simulink model "correlator_core"  (Simulink 7.1)
settings: Solver=ode45  StartTime=0.0  StopTime=10000  RelTol=1e-3
libraries: xbsIndex_r4 x658, cfa_library x168, casper_library_delays x4, casper_library_misc x2
(part 2 of 9)

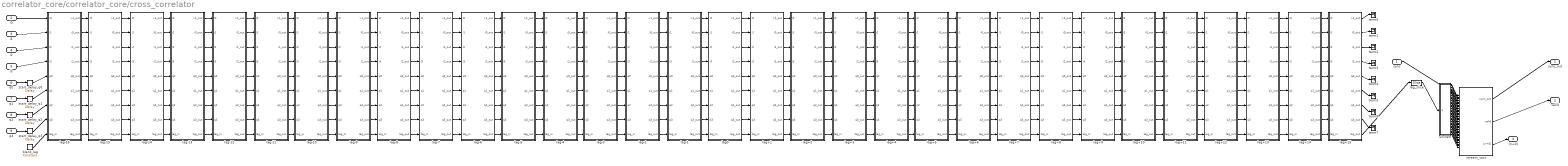
== system correlator_core/correlator_core/cross_correlator ==
  sync : Inport
  i0 : Inport  Port=2
  i1 : Inport  Port=3
  i2 : Inport  Port=4
  i3 : Inport  Port=5
  q0 : Inport  Port=6
  q1 : Inport  Port=7
  q2 : Inport  Port=8
  q3 : Inport  Port=9
  blank_lag : xbsIndex_r4/Constant  arith_type=Unsigned  const=0  n_bits=1  bin_pt=0  explicit_period=on  period=1  equ=P=C  opselect=C  inp2=PCIN>>17  opr=+  inp1=P  carry=CIN  dbl_ovrd=off  block_type=constant
      settings: block_version=11.4
  lag+1 : Subsystem  AncestorBlock=cfa_library/single_lag  mask(single_lag){n_inputs=2, specify_mult=off, mult_spec=Behavioral, specify_add=off, add_spec=Fabric, mult_delay=3, add_delay=2, overall_delay=2, use_2bit=on, shift_q=off, shift_i=on}
      mask prompts: n_inputs "Number of Simultaneous Inputs: (2^?)"; specify_mult "Specify multiplier use (behavioural HDL if not specified)"; mult_spec "Multiplier specification:"; specify_add "Specify adder use (behavioural HDL if not specified)"; add_spec "Adder specification:"; mult_delay "Mult Latency:"; add_delay "Add Latency:"; overall_delay "Overall Latency:"; use_2bit "Use special 2-bit binary encoding"; shift_q "Shift 'q' output"; shift_i "Shift 'i' output"
      mask help: This performs the computations for a single lag. Please use the 'cross_correlator' block to generate a full X-engine.
      mask init:
      | single_lag_init(gcb,...
      |     'n_inputs', n_inputs,...
      |     'specify_mult', specify_mult,...
      |     'mult_spec', mult_spec,...
      |     'specify_add', specify_add,...
      |     'add_spec', add_spec,...
      |     'mult_delay', mult_delay,...
      |     'add_delay', add_delay,...
      |     'overall_delay', overall_delay,...
      |     'use_2bit', use_2bit,...
      |     'shift_q', shift_q,...
      |     'shift_i', shift_i);
      settings: AttributesFormatString=|
      | Use 2-bit: on, Demux: 4,
      | Mult: Behavioral,
      | Add: Fabric
      mask StyleString: edit,checkbox,popup(Behavioral|Core|Embedded),checkbox,popup(Fabric|DSP48),edit,edit,edit,checkbox,checkbox,checkbox
      mask CallbackString:
      | |specify_mult = get_param(gcb,'specify_mult');
      | enables = get_param(gcb, 'MaskEnables');
      | if( strcmp(specify_mult,'off')),
      |     enables{3} = 'off';
      | else,
      |     enables{3} = 'on';
      | end
      | set_param(gcb, 'MaskEnables', enables);
      | ||specify_add = get_param(gcb,'specify_add');
      | enables = get_param(gcb, 'MaskEnables');
      | if( strcmp(specify_add,'off')),
      |     enables{5} = 'off';
      | else,
      |     enables{5} = 'on';
      | end
      | set_param(gcb, 'MaskEnables', enables);
      | |||||||
      mask TabNameString: Basic,Implementation,Implementation,Implementation,Implementation,Implementation,Implementation,Implementation,Basic,Basic,Basic
  lag+10 : Subsystem  AncestorBlock=cfa_library/single_lag  mask(single_lag){n_inputs=2, specify_mult=off, mult_spec=Behavioral, specify_add=off, add_spec=Fabric, mult_delay=3, add_delay=2, overall_delay=2, use_2bit=on, shift_q=off, shift_i=on}
      mask prompts: n_inputs "Number of Simultaneous Inputs: (2^?)"; specify_mult "Specify multiplier use (behavioural HDL if not specified)"; mult_spec "Multiplier specification:"; specify_add "Specify adder use (behavioural HDL if not specified)"; add_spec "Adder specification:"; mult_delay "Mult Latency:"; add_delay "Add Latency:"; overall_delay "Overall Latency:"; use_2bit "Use special 2-bit binary encoding"; shift_q "Shift 'q' output"; shift_i "Shift 'i' output"
      mask help: This performs the computations for a single lag. Please use the 'cross_correlator' block to generate a full X-engine.
      mask init: same as correlator_core/correlator_core/cross_correlator/lag+1
      settings: AttributesFormatString=|
      | Use 2-bit: on, Demux: 4,
      | Mult: Behavioral,
      | Add: Fabric
      mask StyleString: edit,checkbox,popup(Behavioral|Core|Embedded),checkbox,popup(Fabric|DSP48),edit,edit,edit,checkbox,checkbox,checkbox
      mask CallbackString:
      | |specify_mult = get_param(gcb,'specify_mult');
      | enables = get_param(gcb, 'MaskEnables');
      | if( strcmp(specify_mult,'off')),
      |     enables{3} = 'off';
      | else,
      |     enables{3} = 'on';
      | end
      | set_param(gcb, 'MaskEnables', enables);
      | ||specify_add = get_param(gcb,'specify_add');
      | enables = get_param(gcb, 'MaskEnables');
      | if( strcmp(specify_add,'off')),
      |     enables{5} = 'off';
      | else,
      |     enables{5} = 'on';
      | end
      | set_param(gcb, 'MaskEnables', enables);
      | |||||||
      mask TabNameString: Basic,Implementation,Implementation,Implementation,Implementation,Implementation,Implementation,Implementation,Basic,Basic,Basic
  lag+11 : Subsystem  AncestorBlock=cfa_library/single_lag  mask(single_lag){n_inputs=2, specify_mult=off, mult_spec=Behavioral, specify_add=off, add_spec=Fabric, mult_delay=3, add_delay=2, overall_delay=2, use_2bit=on, shift_q=off, shift_i=on}
      mask prompts: n_inputs "Number of Simultaneous Inputs: (2^?)"; specify_mult "Specify multiplier use (behavioural HDL if not specified)"; mult_spec "Multiplier specification:"; specify_add "Specify adder use (behavioural HDL if not specified)"; add_spec "Adder specification:"; mult_delay "Mult Latency:"; add_delay "Add Latency:"; overall_delay "Overall Latency:"; use_2bit "Use special 2-bit binary encoding"; shift_q "Shift 'q' output"; shift_i "Shift 'i' output"
      mask help: This performs the computations for a single lag. Please use the 'cross_correlator' block to generate a full X-engine.
      mask init: same as correlator_core/correlator_core/cross_correlator/lag+1
      settings: AttributesFormatString=|
      | Use 2-bit: on, Demux: 4,
      | Mult: Behavioral,
      | Add: Fabric
      mask StyleString: edit,checkbox,popup(Behavioral|Core|Embedded),checkbox,popup(Fabric|DSP48),edit,edit,edit,checkbox,checkbox,checkbox
      mask CallbackString:
      | |specify_mult = get_param(gcb,'specify_mult');
      | enables = get_param(gcb, 'MaskEnables');
      | if( strcmp(specify_mult,'off')),
      |     enables{3} = 'off';
      | else,
      |     enables{3} = 'on';
      | end
      | set_param(gcb, 'MaskEnables', enables);
      | ||specify_add = get_param(gcb,'specify_add');
      | enables = get_param(gcb, 'MaskEnables');
      | if( strcmp(specify_add,'off')),
      |     enables{5} = 'off';
      | else,
      |     enables{5} = 'on';
      | end
      | set_param(gcb, 'MaskEnables', enables);
      | |||||||
      mask TabNameString: Basic,Implementation,Implementation,Implementation,Implementation,Implementation,Implementation,Implementation,Basic,Basic,Basic
  lag+12 : Subsystem  AncestorBlock=cfa_library/single_lag  mask(single_lag){n_inputs=2, specify_mult=off, mult_spec=Behavioral, specify_add=off, add_spec=Fabric, mult_delay=3, add_delay=2, overall_delay=2, use_2bit=on, shift_q=off, shift_i=on}
      mask prompts: n_inputs "Number of Simultaneous Inputs: (2^?)"; specify_mult "Specify multiplier use (behavioural HDL if not specified)"; mult_spec "Multiplier specification:"; specify_add "Specify adder use (behavioural HDL if not specified)"; add_spec "Adder specification:"; mult_delay "Mult Latency:"; add_delay "Add Latency:"; overall_delay "Overall Latency:"; use_2bit "Use special 2-bit binary encoding"; shift_q "Shift 'q' output"; shift_i "Shift 'i' output"
      mask help: This performs the computations for a single lag. Please use the 'cross_correlator' block to generate a full X-engine.
      mask init: same as correlator_core/correlator_core/cross_correlator/lag+1
      settings: AttributesFormatString=|
      | Use 2-bit: on, Demux: 4,
      | Mult: Behavioral,
      | Add: Fabric
      mask StyleString: edit,checkbox,popup(Behavioral|Core|Embedded),checkbox,popup(Fabric|DSP48),edit,edit,edit,checkbox,checkbox,checkbox
      mask CallbackString:
      | |specify_mult = get_param(gcb,'specify_mult');
      | enables = get_param(gcb, 'MaskEnables');
      | if( strcmp(specify_mult,'off')),
      |     enables{3} = 'off';
      | else,
      |     enables{3} = 'on';
      | end
      | set_param(gcb, 'MaskEnables', enables);
      | ||specify_add = get_param(gcb,'specify_add');
      | enables = get_param(gcb, 'MaskEnables');
      | if( strcmp(specify_add,'off')),
      |     enables{5} = 'off';
      | else,
      |     enables{5} = 'on';
      | end
      | set_param(gcb, 'MaskEnables', enables);
      | |||||||
      mask TabNameString: Basic,Implementation,Implementation,Implementation,Implementation,Implementation,Implementation,Implementation,Basic,Basic,Basic
  lag+13 : Subsystem  AncestorBlock=cfa_library/single_lag  mask(single_lag){n_inputs=2, specify_mult=off, mult_spec=Behavioral, specify_add=off, add_spec=Fabric, mult_delay=3, add_delay=2, overall_delay=2, use_2bit=on, shift_q=off, shift_i=on}
      mask prompts: n_inputs "Number of Simultaneous Inputs: (2^?)"; specify_mult "Specify multiplier use (behavioural HDL if not specified)"; mult_spec "Multiplier specification:"; specify_add "Specify adder use (behavioural HDL if not specified)"; add_spec "Adder specification:"; mult_delay "Mult Latency:"; add_delay "Add Latency:"; overall_delay "Overall Latency:"; use_2bit "Use special 2-bit binary encoding"; shift_q "Shift 'q' output"; shift_i "Shift 'i' output"
      mask help: This performs the computations for a single lag. Please use the 'cross_correlator' block to generate a full X-engine.
      mask init: same as correlator_core/correlator_core/cross_correlator/lag+1
      settings: AttributesFormatString=|
      | Use 2-bit: on, Demux: 4,
      | Mult: Behavioral,
      | Add: Fabric
      mask StyleString: edit,checkbox,popup(Behavioral|Core|Embedded),checkbox,popup(Fabric|DSP48),edit,edit,edit,checkbox,checkbox,checkbox
      mask CallbackString:
      | |specify_mult = get_param(gcb,'specify_mult');
      | enables = get_param(gcb, 'MaskEnables');
      | if( strcmp(specify_mult,'off')),
      |     enables{3} = 'off';
      | else,
      |     enables{3} = 'on';
      | end
      | set_param(gcb, 'MaskEnables', enables);
      | ||specify_add = get_param(gcb,'specify_add');
      | enables = get_param(gcb, 'MaskEnables');
      | if( strcmp(specify_add,'off')),
      |     enables{5} = 'off';
      | else,
      |     enables{5} = 'on';
      | end
      | set_param(gcb, 'MaskEnables', enables);
      | |||||||
      mask TabNameString: Basic,Implementation,Implementation,Implementation,Implementation,Implementation,Implementation,Implementation,Basic,Basic,Basic
  lag+14 : Subsystem  AncestorBlock=cfa_library/single_lag  mask(single_lag){n_inputs=2, specify_mult=off, mult_spec=Behavioral, specify_add=off, add_spec=Fabric, mult_delay=3, add_delay=2, overall_delay=2, use_2bit=on, shift_q=off, shift_i=on}
      mask prompts: n_inputs "Number of Simultaneous Inputs: (2^?)"; specify_mult "Specify multiplier use (behavioural HDL if not specified)"; mult_spec "Multiplier specification:"; specify_add "Specify adder use (behavioural HDL if not specified)"; add_spec "Adder specification:"; mult_delay "Mult Latency:"; add_delay "Add Latency:"; overall_delay "Overall Latency:"; use_2bit "Use special 2-bit binary encoding"; shift_q "Shift 'q' output"; shift_i "Shift 'i' output"
      mask help: This performs the computations for a single lag. Please use the 'cross_correlator' block to generate a full X-engine.
      mask init: same as correlator_core/correlator_core/cross_correlator/lag+1
      settings: AttributesFormatString=|
      | Use 2-bit: on, Demux: 4,
      | Mult: Behavioral,
      | Add: Fabric
      mask StyleString: edit,checkbox,popup(Behavioral|Core|Embedded),checkbox,popup(Fabric|DSP48),edit,edit,edit,checkbox,checkbox,checkbox
      mask CallbackString:
      | |specify_mult = get_param(gcb,'specify_mult');
      | enables = get_param(gcb, 'MaskEnables');
      | if( strcmp(specify_mult,'off')),
      |     enables{3} = 'off';
      | else,
      |     enables{3} = 'on';
      | end
      | set_param(gcb, 'MaskEnables', enables);
      | ||specify_add = get_param(gcb,'specify_add');
      | enables = get_param(gcb, 'MaskEnables');
      | if( strcmp(specify_add,'off')),
      |     enables{5} = 'off';
      | else,
      |     enables{5} = 'on';
      | end
      | set_param(gcb, 'MaskEnables', enables);
      | |||||||
      mask TabNameString: Basic,Implementation,Implementation,Implementation,Implementation,Implementation,Implementation,Implementation,Basic,Basic,Basic
  lag+15 : Subsystem  AncestorBlock=cfa_library/single_lag  mask(single_lag){n_inputs=2, specify_mult=off, mult_spec=Behavioral, specify_add=off, add_spec=Fabric, mult_delay=3, add_delay=2, overall_delay=2, use_2bit=on, shift_q=off, shift_i=on}
      mask prompts: n_inputs "Number of Simultaneous Inputs: (2^?)"; specify_mult "Specify multiplier use (behavioural HDL if not specified)"; mult_spec "Multiplier specification:"; specify_add "Specify adder use (behavioural HDL if not specified)"; add_spec "Adder specification:"; mult_delay "Mult Latency:"; add_delay "Add Latency:"; overall_delay "Overall Latency:"; use_2bit "Use special 2-bit binary encoding"; shift_q "Shift 'q' output"; shift_i "Shift 'i' output"
      mask help: This performs the computations for a single lag. Please use the 'cross_correlator' block to generate a full X-engine.
      mask init: same as correlator_core/correlator_core/cross_correlator/lag+1
      settings: AttributesFormatString=|
      | Use 2-bit: on, Demux: 4,
      | Mult: Behavioral,
      | Add: Fabric
      mask StyleString: edit,checkbox,popup(Behavioral|Core|Embedded),checkbox,popup(Fabric|DSP48),edit,edit,edit,checkbox,checkbox,checkbox
      mask CallbackString:
      | |specify_mult = get_param(gcb,'specify_mult');
      | enables = get_param(gcb, 'MaskEnables');
      | if( strcmp(specify_mult,'off')),
      |     enables{3} = 'off';
      | else,
      |     enables{3} = 'on';
      | end
      | set_param(gcb, 'MaskEnables', enables);
      | ||specify_add = get_param(gcb,'specify_add');
      | enables = get_param(gcb, 'MaskEnables');
      | if( strcmp(specify_add,'off')),
      |     enables{5} = 'off';
      | else,
      |     enables{5} = 'on';
      | end
      | set_param(gcb, 'MaskEnables', enables);
      | |||||||
      mask TabNameString: Basic,Implementation,Implementation,Implementation,Implementation,Implementation,Implementation,Implementation,Basic,Basic,Basic
  lag+2 : Subsystem  AncestorBlock=cfa_library/single_lag  mask(single_lag){n_inputs=2, specify_mult=off, mult_spec=Behavioral, specify_add=off, add_spec=Fabric, mult_delay=3, add_delay=2, overall_delay=2, use_2bit=on, shift_q=off, shift_i=on}
      mask prompts: n_inputs "Number of Simultaneous Inputs: (2^?)"; specify_mult "Specify multiplier use (behavioural HDL if not specified)"; mult_spec "Multiplier specification:"; specify_add "Specify adder use (behavioural HDL if not specified)"; add_spec "Adder specification:"; mult_delay "Mult Latency:"; add_delay "Add Latency:"; overall_delay "Overall Latency:"; use_2bit "Use special 2-bit binary encoding"; shift_q "Shift 'q' output"; shift_i "Shift 'i' output"
      mask help: This performs the computations for a single lag. Please use the 'cross_correlator' block to generate a full X-engine.
      mask init: same as correlator_core/correlator_core/cross_correlator/lag+1
      settings: AttributesFormatString=|
      | Use 2-bit: on, Demux: 4,
      | Mult: Behavioral,
      | Add: Fabric
      mask StyleString: edit,checkbox,popup(Behavioral|Core|Embedded),checkbox,popup(Fabric|DSP48),edit,edit,edit,checkbox,checkbox,checkbox
      mask CallbackString:
      | |specify_mult = get_param(gcb,'specify_mult');
      | enables = get_param(gcb, 'MaskEnables');
      | if( strcmp(specify_mult,'off')),
      |     enables{3} = 'off';
      | else,
      |     enables{3} = 'on';
      | end
      | set_param(gcb, 'MaskEnables', enables);
      | ||specify_add = get_param(gcb,'specify_add');
      | enables = get_param(gcb, 'MaskEnables');
      | if( strcmp(specify_add,'off')),
      |     enables{5} = 'off';
      | else,
      |     enables{5} = 'on';
      | end
      | set_param(gcb, 'MaskEnables', enables);
      | |||||||
      mask TabNameString: Basic,Implementation,Implementation,Implementation,Implementation,Implementation,Implementation,Implementation,Basic,Basic,Basic
  lag+3 : Subsystem  AncestorBlock=cfa_library/single_lag  mask(single_lag){n_inputs=2, specify_mult=off, mult_spec=Behavioral, specify_add=off, add_spec=Fabric, mult_delay=3, add_delay=2, overall_delay=2, use_2bit=on, shift_q=off, shift_i=on}
      mask prompts: n_inputs "Number of Simultaneous Inputs: (2^?)"; specify_mult "Specify multiplier use (behavioural HDL if not specified)"; mult_spec "Multiplier specification:"; specify_add "Specify adder use (behavioural HDL if not specified)"; add_spec "Adder specification:"; mult_delay "Mult Latency:"; add_delay "Add Latency:"; overall_delay "Overall Latency:"; use_2bit "Use special 2-bit binary encoding"; shift_q "Shift 'q' output"; shift_i "Shift 'i' output"
      mask help: This performs the computations for a single lag. Please use the 'cross_correlator' block to generate a full X-engine.
      mask init: same as correlator_core/correlator_core/cross_correlator/lag+1
      settings: AttributesFormatString=|
      | Use 2-bit: on, Demux: 4,
      | Mult: Behavioral,
      | Add: Fabric
      mask StyleString: edit,checkbox,popup(Behavioral|Core|Embedded),checkbox,popup(Fabric|DSP48),edit,edit,edit,checkbox,checkbox,checkbox
      mask CallbackString:
      | |specify_mult = get_param(gcb,'specify_mult');
      | enables = get_param(gcb, 'MaskEnables');
      | if( strcmp(specify_mult,'off')),
      |     enables{3} = 'off';
      | else,
      |     enables{3} = 'on';
      | end
      | set_param(gcb, 'MaskEnables', enables);
      | ||specify_add = get_param(gcb,'specify_add');
      | enables = get_param(gcb, 'MaskEnables');
      | if( strcmp(specify_add,'off')),
      |     enables{5} = 'off';
      | else,
      |     enables{5} = 'on';
      | end
      | set_param(gcb, 'MaskEnables', enables);
      | |||||||
      mask TabNameString: Basic,Implementation,Implementation,Implementation,Implementation,Implementation,Implementation,Implementation,Basic,Basic,Basic
  lag+4 : Subsystem  AncestorBlock=cfa_library/single_lag  mask(single_lag){n_inputs=2, specify_mult=off, mult_spec=Behavioral, specify_add=off, add_spec=Fabric, mult_delay=3, add_delay=2, overall_delay=2, use_2bit=on, shift_q=off, shift_i=on}
      mask prompts: n_inputs "Number of Simultaneous Inputs: (2^?)"; specify_mult "Specify multiplier use (behavioural HDL if not specified)"; mult_spec "Multiplier specification:"; specify_add "Specify adder use (behavioural HDL if not specified)"; add_spec "Adder specification:"; mult_delay "Mult Latency:"; add_delay "Add Latency:"; overall_delay "Overall Latency:"; use_2bit "Use special 2-bit binary encoding"; shift_q "Shift 'q' output"; shift_i "Shift 'i' output"
      mask help: This performs the computations for a single lag. Please use the 'cross_correlator' block to generate a full X-engine.
      mask init: same as correlator_core/correlator_core/cross_correlator/lag+1
      settings: AttributesFormatString=|
      | Use 2-bit: on, Demux: 4,
      | Mult: Behavioral,
      | Add: Fabric
      mask StyleString: edit,checkbox,popup(Behavioral|Core|Embedded),checkbox,popup(Fabric|DSP48),edit,edit,edit,checkbox,checkbox,checkbox
      mask CallbackString:
      | |specify_mult = get_param(gcb,'specify_mult');
      | enables = get_param(gcb, 'MaskEnables');
      | if( strcmp(specify_mult,'off')),
      |     enables{3} = 'off';
      | else,
      |     enables{3} = 'on';
      | end
      | set_param(gcb, 'MaskEnables', enables);
      | ||specify_add = get_param(gcb,'specify_add');
      | enables = get_param(gcb, 'MaskEnables');
      | if( strcmp(specify_add,'off')),
      |     enables{5} = 'off';
      | else,
      |     enables{5} = 'on';
      | end
      | set_param(gcb, 'MaskEnables', enables);
      | |||||||
      mask TabNameString: Basic,Implementation,Implementation,Implementation,Implementation,Implementation,Implementation,Implementation,Basic,Basic,Basic
  lag+5 : Subsystem  AncestorBlock=cfa_library/single_lag  mask(single_lag){n_inputs=2, specify_mult=off, mult_spec=Behavioral, specify_add=off, add_spec=Fabric, mult_delay=3, add_delay=2, overall_delay=2, use_2bit=on, shift_q=off, shift_i=on}
      mask prompts: n_inputs "Number of Simultaneous Inputs: (2^?)"; specify_mult "Specify multiplier use (behavioural HDL if not specified)"; mult_spec "Multiplier specification:"; specify_add "Specify adder use (behavioural HDL if not specified)"; add_spec "Adder specification:"; mult_delay "Mult Latency:"; add_delay "Add Latency:"; overall_delay "Overall Latency:"; use_2bit "Use special 2-bit binary encoding"; shift_q "Shift 'q' output"; shift_i "Shift 'i' output"
      mask help: This performs the computations for a single lag. Please use the 'cross_correlator' block to generate a full X-engine.
      mask init: same as correlator_core/correlator_core/cross_correlator/lag+1
      settings: AttributesFormatString=|
      | Use 2-bit: on, Demux: 4,
      | Mult: Behavioral,
      | Add: Fabric
      mask StyleString: edit,checkbox,popup(Behavioral|Core|Embedded),checkbox,popup(Fabric|DSP48),edit,edit,edit,checkbox,checkbox,checkbox
      mask CallbackString:
      | |specify_mult = get_param(gcb,'specify_mult');
      | enables = get_param(gcb, 'MaskEnables');
      | if( strcmp(specify_mult,'off')),
      |     enables{3} = 'off';
      | else,
      |     enables{3} = 'on';
      | end
      | set_param(gcb, 'MaskEnables', enables);
      | ||specify_add = get_param(gcb,'specify_add');
      | enables = get_param(gcb, 'MaskEnables');
      | if( strcmp(specify_add,'off')),
      |     enables{5} = 'off';
      | else,
      |     enables{5} = 'on';
      | end
      | set_param(gcb, 'MaskEnables', enables);
      | |||||||
      mask TabNameString: Basic,Implementation,Implementation,Implementation,Implementation,Implementation,Implementation,Implementation,Basic,Basic,Basic
  lag+6 : Subsystem  AncestorBlock=cfa_library/single_lag  mask(single_lag){n_inputs=2, specify_mult=off, mult_spec=Behavioral, specify_add=off, add_spec=Fabric, mult_delay=3, add_delay=2, overall_delay=2, use_2bit=on, shift_q=off, shift_i=on}
      mask prompts: n_inputs "Number of Simultaneous Inputs: (2^?)"; specify_mult "Specify multiplier use (behavioural HDL if not specified)"; mult_spec "Multiplier specification:"; specify_add "Specify adder use (behavioural HDL if not specified)"; add_spec "Adder specification:"; mult_delay "Mult Latency:"; add_delay "Add Latency:"; overall_delay "Overall Latency:"; use_2bit "Use special 2-bit binary encoding"; shift_q "Shift 'q' output"; shift_i "Shift 'i' output"
      mask help: This performs the computations for a single lag. Please use the 'cross_correlator' block to generate a full X-engine.
      mask init: same as correlator_core/correlator_core/cross_correlator/lag+1
      settings: AttributesFormatString=|
      | Use 2-bit: on, Demux: 4,
      | Mult: Behavioral,
      | Add: Fabric
      mask StyleString: edit,checkbox,popup(Behavioral|Core|Embedded),checkbox,popup(Fabric|DSP48),edit,edit,edit,checkbox,checkbox,checkbox
      mask CallbackString:
      | |specify_mult = get_param(gcb,'specify_mult');
      | enables = get_param(gcb, 'MaskEnables');
      | if( strcmp(specify_mult,'off')),
      |     enables{3} = 'off';
      | else,
      |     enables{3} = 'on';
      | end
      | set_param(gcb, 'MaskEnables', enables);
      | ||specify_add = get_param(gcb,'specify_add');
      | enables = get_param(gcb, 'MaskEnables');
      | if( strcmp(specify_add,'off')),
      |     enables{5} = 'off';
      | else,
      |     enables{5} = 'on';
      | end
      | set_param(gcb, 'MaskEnables', enables);
      | |||||||
      mask TabNameString: Basic,Implementation,Implementation,Implementation,Implementation,Implementation,Implementation,Implementation,Basic,Basic,Basic
  lag+7 : Subsystem  AncestorBlock=cfa_library/single_lag  mask(single_lag){n_inputs=2, specify_mult=off, mult_spec=Behavioral, specify_add=off, add_spec=Fabric, mult_delay=3, add_delay=2, overall_delay=2, use_2bit=on, shift_q=off, shift_i=on}
      mask prompts: n_inputs "Number of Simultaneous Inputs: (2^?)"; specify_mult "Specify multiplier use (behavioural HDL if not specified)"; mult_spec "Multiplier specification:"; specify_add "Specify adder use (behavioural HDL if not specified)"; add_spec "Adder specification:"; mult_delay "Mult Latency:"; add_delay "Add Latency:"; overall_delay "Overall Latency:"; use_2bit "Use special 2-bit binary encoding"; shift_q "Shift 'q' output"; shift_i "Shift 'i' output"
      mask help: This performs the computations for a single lag. Please use the 'cross_correlator' block to generate a full X-engine.
      mask init: same as correlator_core/correlator_core/cross_correlator/lag+1
      settings: AttributesFormatString=|
      | Use 2-bit: on, Demux: 4,
      | Mult: Behavioral,
      | Add: Fabric
      mask StyleString: edit,checkbox,popup(Behavioral|Core|Embedded),checkbox,popup(Fabric|DSP48),edit,edit,edit,checkbox,checkbox,checkbox
      mask CallbackString:
      | |specify_mult = get_param(gcb,'specify_mult');
      | enables = get_param(gcb, 'MaskEnables');
      | if( strcmp(specify_mult,'off')),
      |     enables{3} = 'off';
      | else,
      |     enables{3} = 'on';
      | end
      | set_param(gcb, 'MaskEnables', enables);
      | ||specify_add = get_param(gcb,'specify_add');
      | enables = get_param(gcb, 'MaskEnables');
      | if( strcmp(specify_add,'off')),
      |     enables{5} = 'off';
      | else,
      |     enables{5} = 'on';
      | end
      | set_param(gcb, 'MaskEnables', enables);
      | |||||||
      mask TabNameString: Basic,Implementation,Implementation,Implementation,Implementation,Implementation,Implementation,Implementation,Basic,Basic,Basic
  lag+8 : Subsystem  AncestorBlock=cfa_library/single_lag  mask(single_lag){n_inputs=2, specify_mult=off, mult_spec=Behavioral, specify_add=off, add_spec=Fabric, mult_delay=3, add_delay=2, overall_delay=2, use_2bit=on, shift_q=off, shift_i=on}
      mask prompts: n_inputs "Number of Simultaneous Inputs: (2^?)"; specify_mult "Specify multiplier use (behavioural HDL if not specified)"; mult_spec "Multiplier specification:"; specify_add "Specify adder use (behavioural HDL if not specified)"; add_spec "Adder specification:"; mult_delay "Mult Latency:"; add_delay "Add Latency:"; overall_delay "Overall Latency:"; use_2bit "Use special 2-bit binary encoding"; shift_q "Shift 'q' output"; shift_i "Shift 'i' output"
      mask help: This performs the computations for a single lag. Please use the 'cross_correlator' block to generate a full X-engine.
      mask init: same as correlator_core/correlator_core/cross_correlator/lag+1
      settings: AttributesFormatString=|
      | Use 2-bit: on, Demux: 4,
      | Mult: Behavioral,
      | Add: Fabric
      mask StyleString: edit,checkbox,popup(Behavioral|Core|Embedded),checkbox,popup(Fabric|DSP48),edit,edit,edit,checkbox,checkbox,checkbox
      mask CallbackString:
      | |specify_mult = get_param(gcb,'specify_mult');
      | enables = get_param(gcb, 'MaskEnables');
      | if( strcmp(specify_mult,'off')),
      |     enables{3} = 'off';
      | else,
      |     enables{3} = 'on';
      | end
      | set_param(gcb, 'MaskEnables', enables);
      | ||specify_add = get_param(gcb,'specify_add');
      | enables = get_param(gcb, 'MaskEnables');
      | if( strcmp(specify_add,'off')),
      |     enables{5} = 'off';
      | else,
      |     enables{5} = 'on';
      | end
      | set_param(gcb, 'MaskEnables', enables);
      | |||||||
      mask TabNameString: Basic,Implementation,Implementation,Implementation,Implementation,Implementation,Implementation,Implementation,Basic,Basic,Basic
  lag+9 : Subsystem  AncestorBlock=cfa_library/single_lag  mask(single_lag){n_inputs=2, specify_mult=off, mult_spec=Behavioral, specify_add=off, add_spec=Fabric, mult_delay=3, add_delay=2, overall_delay=2, use_2bit=on, shift_q=off, shift_i=on}
      mask prompts: n_inputs "Number of Simultaneous Inputs: (2^?)"; specify_mult "Specify multiplier use (behavioural HDL if not specified)"; mult_spec "Multiplier specification:"; specify_add "Specify adder use (behavioural HDL if not specified)"; add_spec "Adder specification:"; mult_delay "Mult Latency:"; add_delay "Add Latency:"; overall_delay "Overall Latency:"; use_2bit "Use special 2-bit binary encoding"; shift_q "Shift 'q' output"; shift_i "Shift 'i' output"
      mask help: This performs the computations for a single lag. Please use the 'cross_correlator' block to generate a full X-engine.
      mask init: same as correlator_core/correlator_core/cross_correlator/lag+1
      settings: AttributesFormatString=|
      | Use 2-bit: on, Demux: 4,
      | Mult: Behavioral,
      | Add: Fabric
      mask StyleString: edit,checkbox,popup(Behavioral|Core|Embedded),checkbox,popup(Fabric|DSP48),edit,edit,edit,checkbox,checkbox,checkbox
      mask CallbackString:
      | |specify_mult = get_param(gcb,'specify_mult');
      | enables = get_param(gcb, 'MaskEnables');
      | if( strcmp(specify_mult,'off')),
      |     enables{3} = 'off';
      | else,
      |     enables{3} = 'on';
      | end
      | set_param(gcb, 'MaskEnables', enables);
      | ||specify_add = get_param(gcb,'specify_add');
      | enables = get_param(gcb, 'MaskEnables');
      | if( strcmp(specify_add,'off')),
      |     enables{5} = 'off';
      | else,
      |     enables{5} = 'on';
      | end
      | set_param(gcb, 'MaskEnables', enables);
      | |||||||
      mask TabNameString: Basic,Implementation,Implementation,Implementation,Implementation,Implementation,Implementation,Implementation,Basic,Basic,Basic
  lag-1 : Subsystem  AncestorBlock=cfa_library/single_lag  mask(single_lag){n_inputs=2, specify_mult=off, mult_spec=Behavioral, specify_add=off, add_spec=Fabric, mult_delay=3, add_delay=2, overall_delay=2, use_2bit=on, shift_q=off, shift_i=on}
      mask prompts: n_inputs "Number of Simultaneous Inputs: (2^?)"; specify_mult "Specify multiplier use (behavioural HDL if not specified)"; mult_spec "Multiplier specification:"; specify_add "Specify adder use (behavioural HDL if not specified)"; add_spec "Adder specification:"; mult_delay "Mult Latency:"; add_delay "Add Latency:"; overall_delay "Overall Latency:"; use_2bit "Use special 2-bit binary encoding"; shift_q "Shift 'q' output"; shift_i "Shift 'i' output"
      mask help: This performs the computations for a single lag. Please use the 'cross_correlator' block to generate a full X-engine.
      mask init: same as correlator_core/correlator_core/cross_correlator/lag+1
      settings: AttributesFormatString=|
      | Use 2-bit: on, Demux: 4,
      | Mult: Behavioral,
      | Add: Fabric
      mask StyleString: edit,checkbox,popup(Behavioral|Core|Embedded),checkbox,popup(Fabric|DSP48),edit,edit,edit,checkbox,checkbox,checkbox
      mask CallbackString:
      | |specify_mult = get_param(gcb,'specify_mult');
      | enables = get_param(gcb, 'MaskEnables');
      | if( strcmp(specify_mult,'off')),
      |     enables{3} = 'off';
      | else,
      |     enables{3} = 'on';
      | end
      | set_param(gcb, 'MaskEnables', enables);
      | ||specify_add = get_param(gcb,'specify_add');
      | enables = get_param(gcb, 'MaskEnables');
      | if( strcmp(specify_add,'off')),
      |     enables{5} = 'off';
      | else,
      |     enables{5} = 'on';
      | end
      | set_param(gcb, 'MaskEnables', enables);
      | |||||||
      mask TabNameString: Basic,Implementation,Implementation,Implementation,Implementation,Implementation,Implementation,Implementation,Basic,Basic,Basic
  lag-10 : Subsystem  AncestorBlock=cfa_library/single_lag  mask(single_lag){n_inputs=2, specify_mult=off, mult_spec=Behavioral, specify_add=off, add_spec=Fabric, mult_delay=3, add_delay=2, overall_delay=2, use_2bit=on, shift_q=off, shift_i=on}
      mask prompts: n_inputs "Number of Simultaneous Inputs: (2^?)"; specify_mult "Specify multiplier use (behavioural HDL if not specified)"; mult_spec "Multiplier specification:"; specify_add "Specify adder use (behavioural HDL if not specified)"; add_spec "Adder specification:"; mult_delay "Mult Latency:"; add_delay "Add Latency:"; overall_delay "Overall Latency:"; use_2bit "Use special 2-bit binary encoding"; shift_q "Shift 'q' output"; shift_i "Shift 'i' output"
      mask help: This performs the computations for a single lag. Please use the 'cross_correlator' block to generate a full X-engine.
      mask init: same as correlator_core/correlator_core/cross_correlator/lag+1
      settings: AttributesFormatString=|
      | Use 2-bit: on, Demux: 4,
      | Mult: Behavioral,
      | Add: Fabric
      mask StyleString: edit,checkbox,popup(Behavioral|Core|Embedded),checkbox,popup(Fabric|DSP48),edit,edit,edit,checkbox,checkbox,checkbox
      mask CallbackString:
      | |specify_mult = get_param(gcb,'specify_mult');
      | enables = get_param(gcb, 'MaskEnables');
      | if( strcmp(specify_mult,'off')),
      |     enables{3} = 'off';
      | else,
      |     enables{3} = 'on';
      | end
      | set_param(gcb, 'MaskEnables', enables);
      | ||specify_add = get_param(gcb,'specify_add');
      | enables = get_param(gcb, 'MaskEnables');
      | if( strcmp(specify_add,'off')),
      |     enables{5} = 'off';
      | else,
      |     enables{5} = 'on';
      | end
      | set_param(gcb, 'MaskEnables', enables);
      | |||||||
      mask TabNameString: Basic,Implementation,Implementation,Implementation,Implementation,Implementation,Implementation,Implementation,Basic,Basic,Basic
  lag-11 : Subsystem  AncestorBlock=cfa_library/single_lag  mask(single_lag){n_inputs=2, specify_mult=off, mult_spec=Behavioral, specify_add=off, add_spec=Fabric, mult_delay=3, add_delay=2, overall_delay=2, use_2bit=on, shift_q=off, shift_i=on}
      mask prompts: n_inputs "Number of Simultaneous Inputs: (2^?)"; specify_mult "Specify multiplier use (behavioural HDL if not specified)"; mult_spec "Multiplier specification:"; specify_add "Specify adder use (behavioural HDL if not specified)"; add_spec "Adder specification:"; mult_delay "Mult Latency:"; add_delay "Add Latency:"; overall_delay "Overall Latency:"; use_2bit "Use special 2-bit binary encoding"; shift_q "Shift 'q' output"; shift_i "Shift 'i' output"
      mask help: This performs the computations for a single lag. Please use the 'cross_correlator' block to generate a full X-engine.
      mask init: same as correlator_core/correlator_core/cross_correlator/lag+1
      settings: AttributesFormatString=|
      | Use 2-bit: on, Demux: 4,
      | Mult: Behavioral,
      | Add: Fabric
      mask StyleString: edit,checkbox,popup(Behavioral|Core|Embedded),checkbox,popup(Fabric|DSP48),edit,edit,edit,checkbox,checkbox,checkbox
      mask CallbackString:
      | |specify_mult = get_param(gcb,'specify_mult');
      | enables = get_param(gcb, 'MaskEnables');
      | if( strcmp(specify_mult,'off')),
      |     enables{3} = 'off';
      | else,
      |     enables{3} = 'on';
      | end
      | set_param(gcb, 'MaskEnables', enables);
      | ||specify_add = get_param(gcb,'specify_add');
      | enables = get_param(gcb, 'MaskEnables');
      | if( strcmp(specify_add,'off')),
      |     enables{5} = 'off';
      | else,
      |     enables{5} = 'on';
      | end
      | set_param(gcb, 'MaskEnables', enables);
      | |||||||
      mask TabNameString: Basic,Implementation,Implementation,Implementation,Implementation,Implementation,Implementation,Implementation,Basic,Basic,Basic
  lag-12 : Subsystem  AncestorBlock=cfa_library/single_lag  mask(single_lag){n_inputs=2, specify_mult=off, mult_spec=Behavioral, specify_add=off, add_spec=Fabric, mult_delay=3, add_delay=2, overall_delay=2, use_2bit=on, shift_q=off, shift_i=on}
      mask prompts: n_inputs "Number of Simultaneous Inputs: (2^?)"; specify_mult "Specify multiplier use (behavioural HDL if not specified)"; mult_spec "Multiplier specification:"; specify_add "Specify adder use (behavioural HDL if not specified)"; add_spec "Adder specification:"; mult_delay "Mult Latency:"; add_delay "Add Latency:"; overall_delay "Overall Latency:"; use_2bit "Use special 2-bit binary encoding"; shift_q "Shift 'q' output"; shift_i "Shift 'i' output"
      mask help: This performs the computations for a single lag. Please use the 'cross_correlator' block to generate a full X-engine.
      mask init: same as correlator_core/correlator_core/cross_correlator/lag+1
      settings: AttributesFormatString=|
      | Use 2-bit: on, Demux: 4,
      | Mult: Behavioral,
      | Add: Fabric
      mask StyleString: edit,checkbox,popup(Behavioral|Core|Embedded),checkbox,popup(Fabric|DSP48),edit,edit,edit,checkbox,checkbox,checkbox
      mask CallbackString:
      | |specify_mult = get_param(gcb,'specify_mult');
      | enables = get_param(gcb, 'MaskEnables');
      | if( strcmp(specify_mult,'off')),
      |     enables{3} = 'off';
      | else,
      |     enables{3} = 'on';
      | end
      | set_param(gcb, 'MaskEnables', enables);
      | ||specify_add = get_param(gcb,'specify_add');
      | enables = get_param(gcb, 'MaskEnables');
      | if( strcmp(specify_add,'off')),
      |     enables{5} = 'off';
      | else,
      |     enables{5} = 'on';
      | end
      | set_param(gcb, 'MaskEnables', enables);
      | |||||||
      mask TabNameString: Basic,Implementation,Implementation,Implementation,Implementation,Implementation,Implementation,Implementation,Basic,Basic,Basic
  lag-13 : Subsystem  AncestorBlock=cfa_library/single_lag  mask(single_lag){n_inputs=2, specify_mult=off, mult_spec=Behavioral, specify_add=off, add_spec=Fabric, mult_delay=3, add_delay=2, overall_delay=2, use_2bit=on, shift_q=off, shift_i=on}
      mask prompts: n_inputs "Number of Simultaneous Inputs: (2^?)"; specify_mult "Specify multiplier use (behavioural HDL if not specified)"; mult_spec "Multiplier specification:"; specify_add "Specify adder use (behavioural HDL if not specified)"; add_spec "Adder specification:"; mult_delay "Mult Latency:"; add_delay "Add Latency:"; overall_delay "Overall Latency:"; use_2bit "Use special 2-bit binary encoding"; shift_q "Shift 'q' output"; shift_i "Shift 'i' output"
      mask help: This performs the computations for a single lag. Please use the 'cross_correlator' block to generate a full X-engine.
      mask init: same as correlator_core/correlator_core/cross_correlator/lag+1
      settings: AttributesFormatString=|
      | Use 2-bit: on, Demux: 4,
      | Mult: Behavioral,
      | Add: Fabric
      mask StyleString: edit,checkbox,popup(Behavioral|Core|Embedded),checkbox,popup(Fabric|DSP48),edit,edit,edit,checkbox,checkbox,checkbox
      mask CallbackString:
      | |specify_mult = get_param(gcb,'specify_mult');
      | enables = get_param(gcb, 'MaskEnables');
      | if( strcmp(specify_mult,'off')),
      |     enables{3} = 'off';
      | else,
      |     enables{3} = 'on';
      | end
      | set_param(gcb, 'MaskEnables', enables);
      | ||specify_add = get_param(gcb,'specify_add');
      | enables = get_param(gcb, 'MaskEnables');
      | if( strcmp(specify_add,'off')),
      |     enables{5} = 'off';
      | else,
      |     enables{5} = 'on';
      | end
      | set_param(gcb, 'MaskEnables', enables);
      | |||||||
      mask TabNameString: Basic,Implementation,Implementation,Implementation,Implementation,Implementation,Implementation,Implementation,Basic,Basic,Basic
  lag-14 : Subsystem  AncestorBlock=cfa_library/single_lag  mask(single_lag){n_inputs=2, specify_mult=off, mult_spec=Behavioral, specify_add=off, add_spec=Fabric, mult_delay=3, add_delay=2, overall_delay=2, use_2bit=on, shift_q=off, shift_i=on}
      mask prompts: n_inputs "Number of Simultaneous Inputs: (2^?)"; specify_mult "Specify multiplier use (behavioural HDL if not specified)"; mult_spec "Multiplier specification:"; specify_add "Specify adder use (behavioural HDL if not specified)"; add_spec "Adder specification:"; mult_delay "Mult Latency:"; add_delay "Add Latency:"; overall_delay "Overall Latency:"; use_2bit "Use special 2-bit binary encoding"; shift_q "Shift 'q' output"; shift_i "Shift 'i' output"
      mask help: This performs the computations for a single lag. Please use the 'cross_correlator' block to generate a full X-engine.
      mask init: same as correlator_core/correlator_core/cross_correlator/lag+1
      settings: AttributesFormatString=|
      | Use 2-bit: on, Demux: 4,
      | Mult: Behavioral,
      | Add: Fabric
      mask StyleString: edit,checkbox,popup(Behavioral|Core|Embedded),checkbox,popup(Fabric|DSP48),edit,edit,edit,checkbox,checkbox,checkbox
      mask CallbackString:
      | |specify_mult = get_param(gcb,'specify_mult');
      | enables = get_param(gcb, 'MaskEnables');
      | if( strcmp(specify_mult,'off')),
      |     enables{3} = 'off';
      | else,
      |     enables{3} = 'on';
      | end
      | set_param(gcb, 'MaskEnables', enables);
      | ||specify_add = get_param(gcb,'specify_add');
      | enables = get_param(gcb, 'MaskEnables');
      | if( strcmp(specify_add,'off')),
      |     enables{5} = 'off';
      | else,
      |     enables{5} = 'on';
      | end
      | set_param(gcb, 'MaskEnables', enables);
      | |||||||
      mask TabNameString: Basic,Implementation,Implementation,Implementation,Implementation,Implementation,Implementation,Implementation,Basic,Basic,Basic
  lag-15 : Subsystem  AncestorBlock=cfa_library/single_lag  mask(single_lag){n_inputs=2, specify_mult=off, mult_spec=Behavioral, specify_add=off, add_spec=Fabric, mult_delay=3, add_delay=2, overall_delay=2, use_2bit=on, shift_q=off, shift_i=on}
      mask prompts: n_inputs "Number of Simultaneous Inputs: (2^?)"; specify_mult "Specify multiplier use (behavioural HDL if not specified)"; mult_spec "Multiplier specification:"; specify_add "Specify adder use (behavioural HDL if not specified)"; add_spec "Adder specification:"; mult_delay "Mult Latency:"; add_delay "Add Latency:"; overall_delay "Overall Latency:"; use_2bit "Use special 2-bit binary encoding"; shift_q "Shift 'q' output"; shift_i "Shift 'i' output"
      mask help: This performs the computations for a single lag. Please use the 'cross_correlator' block to generate a full X-engine.
      mask init: same as correlator_core/correlator_core/cross_correlator/lag+1
      settings: AttributesFormatString=|
      | Use 2-bit: on, Demux: 4,
      | Mult: Behavioral,
      | Add: Fabric
      mask StyleString: edit,checkbox,popup(Behavioral|Core|Embedded),checkbox,popup(Fabric|DSP48),edit,edit,edit,checkbox,checkbox,checkbox
      mask CallbackString:
      | |specify_mult = get_param(gcb,'specify_mult');
      | enables = get_param(gcb, 'MaskEnables');
      | if( strcmp(specify_mult,'off')),
      |     enables{3} = 'off';
      | else,
      |     enables{3} = 'on';
      | end
      | set_param(gcb, 'MaskEnables', enables);
      | ||specify_add = get_param(gcb,'specify_add');
      | enables = get_param(gcb, 'MaskEnables');
      | if( strcmp(specify_add,'off')),
      |     enables{5} = 'off';
      | else,
      |     enables{5} = 'on';
      | end
      | set_param(gcb, 'MaskEnables', enables);
      | |||||||
      mask TabNameString: Basic,Implementation,Implementation,Implementation,Implementation,Implementation,Implementation,Implementation,Basic,Basic,Basic
  lag-16 : Subsystem  AncestorBlock=cfa_library/single_lag  mask(single_lag){n_inputs=2, specify_mult=off, mult_spec=Behavioral, specify_add=off, add_spec=Fabric, mult_delay=3, add_delay=2, overall_delay=2, use_2bit=on, shift_q=off, shift_i=on}
      mask prompts: n_inputs "Number of Simultaneous Inputs: (2^?)"; specify_mult "Specify multiplier use (behavioural HDL if not specified)"; mult_spec "Multiplier specification:"; specify_add "Specify adder use (behavioural HDL if not specified)"; add_spec "Adder specification:"; mult_delay "Mult Latency:"; add_delay "Add Latency:"; overall_delay "Overall Latency:"; use_2bit "Use special 2-bit binary encoding"; shift_q "Shift 'q' output"; shift_i "Shift 'i' output"
      mask help: This performs the computations for a single lag. Please use the 'cross_correlator' block to generate a full X-engine.
      mask init: same as correlator_core/correlator_core/cross_correlator/lag+1
      settings: AttributesFormatString=|
      | Use 2-bit: on, Demux: 4,
      | Mult: Behavioral,
      | Add: Fabric
      mask StyleString: edit,checkbox,popup(Behavioral|Core|Embedded),checkbox,popup(Fabric|DSP48),edit,edit,edit,checkbox,checkbox,checkbox
      mask CallbackString:
      | |specify_mult = get_param(gcb,'specify_mult');
      | enables = get_param(gcb, 'MaskEnables');
      | if( strcmp(specify_mult,'off')),
      |     enables{3} = 'off';
      | else,
      |     enables{3} = 'on';
      | end
      | set_param(gcb, 'MaskEnables', enables);
      | ||specify_add = get_param(gcb,'specify_add');
      | enables = get_param(gcb, 'MaskEnables');
      | if( strcmp(specify_add,'off')),
      |     enables{5} = 'off';
      | else,
      |     enables{5} = 'on';
      | end
      | set_param(gcb, 'MaskEnables', enables);
      | |||||||
      mask TabNameString: Basic,Implementation,Implementation,Implementation,Implementation,Implementation,Implementation,Implementation,Basic,Basic,Basic
  lag-2 : Subsystem  AncestorBlock=cfa_library/single_lag  mask(single_lag){n_inputs=2, specify_mult=off, mult_spec=Behavioral, specify_add=off, add_spec=Fabric, mult_delay=3, add_delay=2, overall_delay=2, use_2bit=on, shift_q=off, shift_i=on}
      mask prompts: n_inputs "Number of Simultaneous Inputs: (2^?)"; specify_mult "Specify multiplier use (behavioural HDL if not specified)"; mult_spec "Multiplier specification:"; specify_add "Specify adder use (behavioural HDL if not specified)"; add_spec "Adder specification:"; mult_delay "Mult Latency:"; add_delay "Add Latency:"; overall_delay "Overall Latency:"; use_2bit "Use special 2-bit binary encoding"; shift_q "Shift 'q' output"; shift_i "Shift 'i' output"
      mask help: This performs the computations for a single lag. Please use the 'cross_correlator' block to generate a full X-engine.
      mask init: same as correlator_core/correlator_core/cross_correlator/lag+1
      settings: AttributesFormatString=|
      | Use 2-bit: on, Demux: 4,
      | Mult: Behavioral,
      | Add: Fabric
      mask StyleString: edit,checkbox,popup(Behavioral|Core|Embedded),checkbox,popup(Fabric|DSP48),edit,edit,edit,checkbox,checkbox,checkbox
      mask CallbackString:
      | |specify_mult = get_param(gcb,'specify_mult');
      | enables = get_param(gcb, 'MaskEnables');
      | if( strcmp(specify_mult,'off')),
      |     enables{3} = 'off';
      | else,
      |     enables{3} = 'on';
      | end
      | set_param(gcb, 'MaskEnables', enables);
      | ||specify_add = get_param(gcb,'specify_add');
      | enables = get_param(gcb, 'MaskEnables');
      | if( strcmp(specify_add,'off')),
      |     enables{5} = 'off';
      | else,
      |     enables{5} = 'on';
      | end
      | set_param(gcb, 'MaskEnables', enables);
      | |||||||
      mask TabNameString: Basic,Implementation,Implementation,Implementation,Implementation,Implementation,Implementation,Implementation,Basic,Basic,Basic
  lag-3 : Subsystem  AncestorBlock=cfa_library/single_lag  mask(single_lag){n_inputs=2, specify_mult=off, mult_spec=Behavioral, specify_add=off, add_spec=Fabric, mult_delay=3, add_delay=2, overall_delay=2, use_2bit=on, shift_q=off, shift_i=on}
      mask prompts: n_inputs "Number of Simultaneous Inputs: (2^?)"; specify_mult "Specify multiplier use (behavioural HDL if not specified)"; mult_spec "Multiplier specification:"; specify_add "Specify adder use (behavioural HDL if not specified)"; add_spec "Adder specification:"; mult_delay "Mult Latency:"; add_delay "Add Latency:"; overall_delay "Overall Latency:"; use_2bit "Use special 2-bit binary encoding"; shift_q "Shift 'q' output"; shift_i "Shift 'i' output"
      mask help: This performs the computations for a single lag. Please use the 'cross_correlator' block to generate a full X-engine.
      mask init: same as correlator_core/correlator_core/cross_correlator/lag+1
      settings: AttributesFormatString=|
      | Use 2-bit: on, Demux: 4,
      | Mult: Behavioral,
      | Add: Fabric
      mask StyleString: edit,checkbox,popup(Behavioral|Core|Embedded),checkbox,popup(Fabric|DSP48),edit,edit,edit,checkbox,checkbox,checkbox
      mask CallbackString:
      | |specify_mult = get_param(gcb,'specify_mult');
      | enables = get_param(gcb, 'MaskEnables');
      | if( strcmp(specify_mult,'off')),
      |     enables{3} = 'off';
      | else,
      |     enables{3} = 'on';
      | end
      | set_param(gcb, 'MaskEnables', enables);
      | ||specify_add = get_param(gcb,'specify_add');
      | enables = get_param(gcb, 'MaskEnables');
      | if( strcmp(specify_add,'off')),
      |     enables{5} = 'off';
      | else,
      |     enables{5} = 'on';
      | end
      | set_param(gcb, 'MaskEnables', enables);
      | |||||||
      mask TabNameString: Basic,Implementation,Implementation,Implementation,Implementation,Implementation,Implementation,Implementation,Basic,Basic,Basic
  lag-4 : Subsystem  AncestorBlock=cfa_library/single_lag  mask(single_lag){n_inputs=2, specify_mult=off, mult_spec=Behavioral, specify_add=off, add_spec=Fabric, mult_delay=3, add_delay=2, overall_delay=2, use_2bit=on, shift_q=off, shift_i=on}
      mask prompts: n_inputs "Number of Simultaneous Inputs: (2^?)"; specify_mult "Specify multiplier use (behavioural HDL if not specified)"; mult_spec "Multiplier specification:"; specify_add "Specify adder use (behavioural HDL if not specified)"; add_spec "Adder specification:"; mult_delay "Mult Latency:"; add_delay "Add Latency:"; overall_delay "Overall Latency:"; use_2bit "Use special 2-bit binary encoding"; shift_q "Shift 'q' output"; shift_i "Shift 'i' output"
      mask help: This performs the computations for a single lag. Please use the 'cross_correlator' block to generate a full X-engine.
      mask init: same as correlator_core/correlator_core/cross_correlator/lag+1
      settings: AttributesFormatString=|
      | Use 2-bit: on, Demux: 4,
      | Mult: Behavioral,
      | Add: Fabric
      mask StyleString: edit,checkbox,popup(Behavioral|Core|Embedded),checkbox,popup(Fabric|DSP48),edit,edit,edit,checkbox,checkbox,checkbox
      mask CallbackString:
      | |specify_mult = get_param(gcb,'specify_mult');
      | enables = get_param(gcb, 'MaskEnables');
      | if( strcmp(specify_mult,'off')),
      |     enables{3} = 'off';
      | else,
      |     enables{3} = 'on';
      | end
      | set_param(gcb, 'MaskEnables', enables);
      | ||specify_add = get_param(gcb,'specify_add');
      | enables = get_param(gcb, 'MaskEnables');
      | if( strcmp(specify_add,'off')),
      |     enables{5} = 'off';
      | else,
      |     enables{5} = 'on';
      | end
      | set_param(gcb, 'MaskEnables', enables);
      | |||||||
      mask TabNameString: Basic,Implementation,Implementation,Implementation,Implementation,Implementation,Implementation,Implementation,Basic,Basic,Basic
  lag-5 : Subsystem  AncestorBlock=cfa_library/single_lag  mask(single_lag){n_inputs=2, specify_mult=off, mult_spec=Behavioral, specify_add=off, add_spec=Fabric, mult_delay=3, add_delay=2, overall_delay=2, use_2bit=on, shift_q=off, shift_i=on}
      mask prompts: n_inputs "Number of Simultaneous Inputs: (2^?)"; specify_mult "Specify multiplier use (behavioural HDL if not specified)"; mult_spec "Multiplier specification:"; specify_add "Specify adder use (behavioural HDL if not specified)"; add_spec "Adder specification:"; mult_delay "Mult Latency:"; add_delay "Add Latency:"; overall_delay "Overall Latency:"; use_2bit "Use special 2-bit binary encoding"; shift_q "Shift 'q' output"; shift_i "Shift 'i' output"
      mask help: This performs the computations for a single lag. Please use the 'cross_correlator' block to generate a full X-engine.
      mask init: same as correlator_core/correlator_core/cross_correlator/lag+1
      settings: AttributesFormatString=|
      | Use 2-bit: on, Demux: 4,
      | Mult: Behavioral,
      | Add: Fabric
      mask StyleString: edit,checkbox,popup(Behavioral|Core|Embedded),checkbox,popup(Fabric|DSP48),edit,edit,edit,checkbox,checkbox,checkbox
      mask CallbackString:
      | |specify_mult = get_param(gcb,'specify_mult');
      | enables = get_param(gcb, 'MaskEnables');
      | if( strcmp(specify_mult,'off')),
      |     enables{3} = 'off';
      | else,
      |     enables{3} = 'on';
      | end
      | set_param(gcb, 'MaskEnables', enables);
      | ||specify_add = get_param(gcb,'specify_add');
      | enables = get_param(gcb, 'MaskEnables');
      | if( strcmp(specify_add,'off')),
      |     enables{5} = 'off';
      | else,
      |     enables{5} = 'on';
      | end
      | set_param(gcb, 'MaskEnables', enables);
      | |||||||
      mask TabNameString: Basic,Implementation,Implementation,Implementation,Implementation,Implementation,Implementation,Implementation,Basic,Basic,Basic
  lag-6 : Subsystem  AncestorBlock=cfa_library/single_lag  mask(single_lag){n_inputs=2, specify_mult=off, mult_spec=Behavioral, specify_add=off, add_spec=Fabric, mult_delay=3, add_delay=2, overall_delay=2, use_2bit=on, shift_q=off, shift_i=on}
      mask prompts: n_inputs "Number of Simultaneous Inputs: (2^?)"; specify_mult "Specify multiplier use (behavioural HDL if not specified)"; mult_spec "Multiplier specification:"; specify_add "Specify adder use (behavioural HDL if not specified)"; add_spec "Adder specification:"; mult_delay "Mult Latency:"; add_delay "Add Latency:"; overall_delay "Overall Latency:"; use_2bit "Use special 2-bit binary encoding"; shift_q "Shift 'q' output"; shift_i "Shift 'i' output"
      mask help: This performs the computations for a single lag. Please use the 'cross_correlator' block to generate a full X-engine.
      mask init: same as correlator_core/correlator_core/cross_correlator/lag+1
      settings: AttributesFormatString=|
      | Use 2-bit: on, Demux: 4,
      | Mult: Behavioral,
      | Add: Fabric
      mask StyleString: edit,checkbox,popup(Behavioral|Core|Embedded),checkbox,popup(Fabric|DSP48),edit,edit,edit,checkbox,checkbox,checkbox
      mask CallbackString:
      | |specify_mult = get_param(gcb,'specify_mult');
      | enables = get_param(gcb, 'MaskEnables');
      | if( strcmp(specify_mult,'off')),
      |     enables{3} = 'off';
      | else,
      |     enables{3} = 'on';
      | end
      | set_param(gcb, 'MaskEnables', enables);
      | ||specify_add = get_param(gcb,'specify_add');
      | enables = get_param(gcb, 'MaskEnables');
      | if( strcmp(specify_add,'off')),
      |     enables{5} = 'off';
      | else,
      |     enables{5} = 'on';
      | end
      | set_param(gcb, 'MaskEnables', enables);
      | |||||||
      mask TabNameString: Basic,Implementation,Implementation,Implementation,Implementation,Implementation,Implementation,Implementation,Basic,Basic,Basic
  lag-7 : Subsystem  AncestorBlock=cfa_library/single_lag  mask(single_lag){n_inputs=2, specify_mult=off, mult_spec=Behavioral, specify_add=off, add_spec=Fabric, mult_delay=3, add_delay=2, overall_delay=2, use_2bit=on, shift_q=off, shift_i=on}
      mask prompts: n_inputs "Number of Simultaneous Inputs: (2^?)"; specify_mult "Specify multiplier use (behavioural HDL if not specified)"; mult_spec "Multiplier specification:"; specify_add "Specify adder use (behavioural HDL if not specified)"; add_spec "Adder specification:"; mult_delay "Mult Latency:"; add_delay "Add Latency:"; overall_delay "Overall Latency:"; use_2bit "Use special 2-bit binary encoding"; shift_q "Shift 'q' output"; shift_i "Shift 'i' output"
      mask help: This performs the computations for a single lag. Please use the 'cross_correlator' block to generate a full X-engine.
      mask init: same as correlator_core/correlator_core/cross_correlator/lag+1
      settings: AttributesFormatString=|
      | Use 2-bit: on, Demux: 4,
      | Mult: Behavioral,
      | Add: Fabric
      mask StyleString: edit,checkbox,popup(Behavioral|Core|Embedded),checkbox,popup(Fabric|DSP48),edit,edit,edit,checkbox,checkbox,checkbox
      mask CallbackString:
      | |specify_mult = get_param(gcb,'specify_mult');
      | enables = get_param(gcb, 'MaskEnables');
      | if( strcmp(specify_mult,'off')),
      |     enables{3} = 'off';
      | else,
      |     enables{3} = 'on';
      | end
      | set_param(gcb, 'MaskEnables', enables);
      | ||specify_add = get_param(gcb,'specify_add');
      | enables = get_param(gcb, 'MaskEnables');
      | if( strcmp(specify_add,'off')),
      |     enables{5} = 'off';
      | else,
      |     enables{5} = 'on';
      | end
      | set_param(gcb, 'MaskEnables', enables);
      | |||||||
      mask TabNameString: Basic,Implementation,Implementation,Implementation,Implementation,Implementation,Implementation,Implementation,Basic,Basic,Basic
  lag-8 : Subsystem  AncestorBlock=cfa_library/single_lag  mask(single_lag){n_inputs=2, specify_mult=off, mult_spec=Behavioral, specify_add=off, add_spec=Fabric, mult_delay=3, add_delay=2, overall_delay=2, use_2bit=on, shift_q=off, shift_i=on}
      mask prompts: n_inputs "Number of Simultaneous Inputs: (2^?)"; specify_mult "Specify multiplier use (behavioural HDL if not specified)"; mult_spec "Multiplier specification:"; specify_add "Specify adder use (behavioural HDL if not specified)"; add_spec "Adder specification:"; mult_delay "Mult Latency:"; add_delay "Add Latency:"; overall_delay "Overall Latency:"; use_2bit "Use special 2-bit binary encoding"; shift_q "Shift 'q' output"; shift_i "Shift 'i' output"
      mask help: This performs the computations for a single lag. Please use the 'cross_correlator' block to generate a full X-engine.
      mask init: same as correlator_core/correlator_core/cross_correlator/lag+1
      settings: AttributesFormatString=|
      | Use 2-bit: on, Demux: 4,
      | Mult: Behavioral,
      | Add: Fabric
      mask StyleString: edit,checkbox,popup(Behavioral|Core|Embedded),checkbox,popup(Fabric|DSP48),edit,edit,edit,checkbox,checkbox,checkbox
      mask CallbackString:
      | |specify_mult = get_param(gcb,'specify_mult');
      | enables = get_param(gcb, 'MaskEnables');
      | if( strcmp(specify_mult,'off')),
      |     enables{3} = 'off';
      | else,
      |     enables{3} = 'on';
      | end
      | set_param(gcb, 'MaskEnables', enables);
      | ||specify_add = get_param(gcb,'specify_add');
      | enables = get_param(gcb, 'MaskEnables');
      | if( strcmp(specify_add,'off')),
      |     enables{5} = 'off';
      | else,
      |     enables{5} = 'on';
      | end
      | set_param(gcb, 'MaskEnables', enables);
      | |||||||
      mask TabNameString: Basic,Implementation,Implementation,Implementation,Implementation,Implementation,Implementation,Implementation,Basic,Basic,Basic
  lag-9 : Subsystem  AncestorBlock=cfa_library/single_lag  mask(single_lag){n_inputs=2, specify_mult=off, mult_spec=Behavioral, specify_add=off, add_spec=Fabric, mult_delay=3, add_delay=2, overall_delay=2, use_2bit=on, shift_q=off, shift_i=on}
      mask prompts: n_inputs "Number of Simultaneous Inputs: (2^?)"; specify_mult "Specify multiplier use (behavioural HDL if not specified)"; mult_spec "Multiplier specification:"; specify_add "Specify adder use (behavioural HDL if not specified)"; add_spec "Adder specification:"; mult_delay "Mult Latency:"; add_delay "Add Latency:"; overall_delay "Overall Latency:"; use_2bit "Use special 2-bit binary encoding"; shift_q "Shift 'q' output"; shift_i "Shift 'i' output"
      mask help: This performs the computations for a single lag. Please use the 'cross_correlator' block to generate a full X-engine.
      mask init: same as correlator_core/correlator_core/cross_correlator/lag+1
      settings: AttributesFormatString=|
      | Use 2-bit: on, Demux: 4,
      | Mult: Behavioral,
      | Add: Fabric
      mask StyleString: edit,checkbox,popup(Behavioral|Core|Embedded),checkbox,popup(Fabric|DSP48),edit,edit,edit,checkbox,checkbox,checkbox
      mask CallbackString:
      | |specify_mult = get_param(gcb,'specify_mult');
      | enables = get_param(gcb, 'MaskEnables');
      | if( strcmp(specify_mult,'off')),
      |     enables{3} = 'off';
      | else,
      |     enables{3} = 'on';
      | end
      | set_param(gcb, 'MaskEnables', enables);
      | ||specify_add = get_param(gcb,'specify_add');
      | enables = get_param(gcb, 'MaskEnables');
      | if( strcmp(specify_add,'off')),
      |     enables{5} = 'off';
      | else,
      |     enables{5} = 'on';
      | end
      | set_param(gcb, 'MaskEnables', enables);
      | |||||||
      mask TabNameString: Basic,Implementation,Implementation,Implementation,Implementation,Implementation,Implementation,Implementation,Basic,Basic,Basic
  lag0 : Subsystem  AncestorBlock=cfa_library/single_lag  mask(single_lag){n_inputs=2, specify_mult=off, mult_spec=Behavioral, specify_add=off, add_spec=Fabric, mult_delay=3, add_delay=2, overall_delay=2, use_2bit=on, shift_q=off, shift_i=on}
      mask prompts: n_inputs "Number of Simultaneous Inputs: (2^?)"; specify_mult "Specify multiplier use (behavioural HDL if not specified)"; mult_spec "Multiplier specification:"; specify_add "Specify adder use (behavioural HDL if not specified)"; add_spec "Adder specification:"; mult_delay "Mult Latency:"; add_delay "Add Latency:"; overall_delay "Overall Latency:"; use_2bit "Use special 2-bit binary encoding"; shift_q "Shift 'q' output"; shift_i "Shift 'i' output"
      mask help: This performs the computations for a single lag. Please use the 'cross_correlator' block to generate a full X-engine.
      mask init: same as correlator_core/correlator_core/cross_correlator/lag+1
      settings: AttributesFormatString=|
      | Use 2-bit: on, Demux: 4,
      | Mult: Behavioral,
      | Add: Fabric
      mask StyleString: edit,checkbox,popup(Behavioral|Core|Embedded),checkbox,popup(Fabric|DSP48),edit,edit,edit,checkbox,checkbox,checkbox
      mask CallbackString:
      | |specify_mult = get_param(gcb,'specify_mult');
      | enables = get_param(gcb, 'MaskEnables');
      | if( strcmp(specify_mult,'off')),
      |     enables{3} = 'off';
      | else,
      |     enables{3} = 'on';
      | end
      | set_param(gcb, 'MaskEnables', enables);
      | ||specify_add = get_param(gcb,'specify_add');
      | enables = get_param(gcb, 'MaskEnables');
      | if( strcmp(specify_add,'off')),
      |     enables{5} = 'off';
      | else,
      |     enables{5} = 'on';
      | end
      | set_param(gcb, 'MaskEnables', enables);
      | |||||||
      mask TabNameString: Basic,Implementation,Implementation,Implementation,Implementation,Implementation,Implementation,Implementation,Basic,Basic,Basic
  lag_slice : xbsIndex_r4/Slice  nbits=224  boolean_output=off  mode=Lower Bit Location + Width  bit1=0  base1=MSB of Input  bit0=0  base0=LSB of Input  dbl_ovrd=off  block_type=slice
  start_delay_q{0..3} (4 alike) : xbsIndex_r4/Delay  en=off  latency=4  dbl_ovrd=off  reg_retiming=off  block_type=delay
      start_delay_q0 settings: block_version=11.4
      start_delay_q1 settings: block_version=11.4
  stream_vacc : Subsystem  AncestorBlock=cfa_library/stream_vacc  mask(stream_vacc){vector_len=5, input_bit_width=7, input_bin_pt=0, samples_out=0, output_bit_width=11, output_bin_pt=0, quantization=Truncate, overflow=Wrap, specify_add=off, add_spec=Fabric, add_delay=1}
      mask prompts: vector_len "Vector Length: (2^?)"; input_bit_width "Input Bit Width:"; input_bin_pt "Input Binary Point:"; samples_out "Number of Simultaneous Outputs: (2^?)"; output_bit_width "Output Bit Width:"; output_bin_pt "Output Binary Point:"; quantization "Quantization Behavior:"; overflow "Overflow Behavior:"; specify_add "Specify adder use (behavioural HDL if not specified)"; add_spec "Adder specification:"; add_delay "Add Latency:"
      mask help: This block implements the second stage adder for the cross_correlator block.
      mask init:
      | stream_vacc_init(gcb,...
      |     'vector_len', vector_len,...
      |     'input_bit_width', input_bit_width,...
      |     'input_bin_pt', input_bin_pt,...
      |     'samples_out', samples_out,...
      |     'output_bit_width', output_bit_width,...
      |     'output_bin_pt', output_bin_pt,...
      |     'quantization', quantization,...
      |     'overflow', overflow,...
      |     'specify_add', specify_add,...
      |     'add_spec', add_spec,...
      |     'add_delay', add_delay);
      settings: AttributesFormatString=|
      | 32=>1 samples
      | Accumulate
      mask StyleString: edit,edit,edit,edit,edit,edit,popup(Truncate|Round  (unbiased: +/- Inf)),popup(Wrap|Saturate|Flag as error),checkbox,popup(Fabric|DSP48),edit
      mask CallbackString:
      | |||vector_len = str2num(get_param(gcb, 'vector_len'));
      | samples_out = str2num(get_param(gcb, 'samples_out'));
      | 
      | if vector_len<samples_out,
      |     error('Number of parallel streams must be greater than or equal to the vector length!');
      | end|||||specify_add = get_param(gcb,'specify_add');
      | visibs = get_param(gcb, 'MaskVisibilities');
      | if( strcmp(specify_add,'off')),
      |     visibs{10} = 'off';
      | else
      |     visibs{10} = 'on';
      | end
      | set_param(gcb, 'MaskVisibilities', visibs);||
  term{0..7} (8 alike) : Terminator
  uncram : Subsystem  AncestorBlock=gavrt_library/uncram  mask(uncram){num_slice=32, slice_width=7, bin_pt=0, arith_type=0}
      mask prompts: num_slice "Number of slices"; slice_width "Slice Width"; bin_pt "Output Binary Point"; arith_type "Output Arithmetic Type (0=Unsigned, 1=Signed)"
      mask help: Takes a concatenated input and slices it up into even pieces and reinterprets them as signed fixed point numbers with a given binary point.
      mask init:
      | uncram_init(gcb, ...
      |     'num_slice', num_slice, ...
      |     'slice_width', slice_width, ...
      |     'bin_pt', bin_pt, ...
      |     'arith_type', arith_type);
      settings: AttributesFormatString=UFix_7_0
  sync_out : Outport
  valid : Outport  Port=2
  "[n+0]" : Outport  Port=3
  wires:
  q0/1 -> start_delay_q0/1
  q1/1 -> start_delay_q1/1
  q2/1 -> start_delay_q2/1
  q3/1 -> start_delay_q3/1
  blank_lag/1 -> lag-16/9(lag_in)
  i0/1 -> lag-16/1(i0)
  start_delay_q0/1 -> lag-16/5(q0)
  i1/1 -> lag-16/2(i1)
  start_delay_q1/1 -> lag-16/6(q1)
  i2/1 -> lag-16/3(i2)
  start_delay_q2/1 -> lag-16/7(q2)
  i3/1 -> lag-16/4(i3)
  start_delay_q3/1 -> lag-16/8(q3)
  lag-16/1(i-1_out) -> lag-15/1(i0)
  lag-16/2(i0_out) -> lag-15/2(i1)
  lag-16/3(i1_out) -> lag-15/3(i2)
  lag-16/4(i2_out) -> lag-15/4(i3)
  lag-16/5(q0_out) -> lag-15/5(q0)
  lag-16/6(q1_out) -> lag-15/6(q1)
  lag-16/7(q2_out) -> lag-15/7(q2)
  lag-16/8(q3_out) -> lag-15/8(q3)
  lag-16/9(lag_out) -> lag-15/9(lag_in)
  lag-15/1(i-1_out) -> lag-14/1(i0)
  lag-15/2(i0_out) -> lag-14/2(i1)
  lag-15/3(i1_out) -> lag-14/3(i2)
  lag-15/4(i2_out) -> lag-14/4(i3)
  lag-15/5(q0_out) -> lag-14/5(q0)
  lag-15/6(q1_out) -> lag-14/6(q1)
  lag-15/7(q2_out) -> lag-14/7(q2)
  lag-15/8(q3_out) -> lag-14/8(q3)
  lag-15/9(lag_out) -> lag-14/9(lag_in)
  lag-14/1(i-1_out) -> lag-13/1(i0)
  lag-14/2(i0_out) -> lag-13/2(i1)
  lag-14/3(i1_out) -> lag-13/3(i2)
  lag-14/4(i2_out) -> lag-13/4(i3)
  lag-14/5(q0_out) -> lag-13/5(q0)
  lag-14/6(q1_out) -> lag-13/6(q1)
  lag-14/7(q2_out) -> lag-13/7(q2)
  lag-14/8(q3_out) -> lag-13/8(q3)
  lag-14/9(lag_out) -> lag-13/9(lag_in)
  lag-13/1(i-1_out) -> lag-12/1(i0)
  lag-13/2(i0_out) -> lag-12/2(i1)
  lag-13/3(i1_out) -> lag-12/3(i2)
  lag-13/4(i2_out) -> lag-12/4(i3)
  lag-13/5(q0_out) -> lag-12/5(q0)
  lag-13/6(q1_out) -> lag-12/6(q1)
  lag-13/7(q2_out) -> lag-12/7(q2)
  lag-13/8(q3_out) -> lag-12/8(q3)
  lag-13/9(lag_out) -> lag-12/9(lag_in)
  lag-12/1(i-1_out) -> lag-11/1(i0)
  lag-12/2(i0_out) -> lag-11/2(i1)
  lag-12/3(i1_out) -> lag-11/3(i2)
  lag-12/4(i2_out) -> lag-11/4(i3)
  lag-12/5(q0_out) -> lag-11/5(q0)
  lag-12/6(q1_out) -> lag-11/6(q1)
  lag-12/7(q2_out) -> lag-11/7(q2)
  lag-12/8(q3_out) -> lag-11/8(q3)
  lag-12/9(lag_out) -> lag-11/9(lag_in)
  lag-11/1(i-1_out) -> lag-10/1(i0)
  lag-11/2(i0_out) -> lag-10/2(i1)
  lag-11/3(i1_out) -> lag-10/3(i2)
  lag-11/4(i2_out) -> lag-10/4(i3)
  lag-11/5(q0_out) -> lag-10/5(q0)
  lag-11/6(q1_out) -> lag-10/6(q1)
  lag-11/7(q2_out) -> lag-10/7(q2)
  lag-11/8(q3_out) -> lag-10/8(q3)
  lag-11/9(lag_out) -> lag-10/9(lag_in)
  lag-10/1(i-1_out) -> lag-9/1(i0)
  lag-10/2(i0_out) -> lag-9/2(i1)
  lag-10/3(i1_out) -> lag-9/3(i2)
  lag-10/4(i2_out) -> lag-9/4(i3)
  lag-10/5(q0_out) -> lag-9/5(q0)
  lag-10/6(q1_out) -> lag-9/6(q1)
  lag-10/7(q2_out) -> lag-9/7(q2)
  lag-10/8(q3_out) -> lag-9/8(q3)
  lag-10/9(lag_out) -> lag-9/9(lag_in)
  lag-9/1(i-1_out) -> lag-8/1(i0)
  lag-9/2(i0_out) -> lag-8/2(i1)
  lag-9/3(i1_out) -> lag-8/3(i2)
  lag-9/4(i2_out) -> lag-8/4(i3)
  lag-9/5(q0_out) -> lag-8/5(q0)
  lag-9/6(q1_out) -> lag-8/6(q1)
  lag-9/7(q2_out) -> lag-8/7(q2)
  lag-9/8(q3_out) -> lag-8/8(q3)
  lag-9/9(lag_out) -> lag-8/9(lag_in)
  lag-8/1(i-1_out) -> lag-7/1(i0)
  lag-8/2(i0_out) -> lag-7/2(i1)
  lag-8/3(i1_out) -> lag-7/3(i2)
  lag-8/4(i2_out) -> lag-7/4(i3)
  lag-8/5(q0_out) -> lag-7/5(q0)
  lag-8/6(q1_out) -> lag-7/6(q1)
  lag-8/7(q2_out) -> lag-7/7(q2)
  lag-8/8(q3_out) -> lag-7/8(q3)
  lag-8/9(lag_out) -> lag-7/9(lag_in)
  lag-7/1(i-1_out) -> lag-6/1(i0)
  lag-7/2(i0_out) -> lag-6/2(i1)
  lag-7/3(i1_out) -> lag-6/3(i2)
  lag-7/4(i2_out) -> lag-6/4(i3)
  lag-7/5(q0_out) -> lag-6/5(q0)
  lag-7/6(q1_out) -> lag-6/6(q1)
  lag-7/7(q2_out) -> lag-6/7(q2)
  lag-7/8(q3_out) -> lag-6/8(q3)
  lag-7/9(lag_out) -> lag-6/9(lag_in)
  lag-6/1(i-1_out) -> lag-5/1(i0)
  lag-6/2(i0_out) -> lag-5/2(i1)
  lag-6/3(i1_out) -> lag-5/3(i2)
  lag-6/4(i2_out) -> lag-5/4(i3)
  lag-6/5(q0_out) -> lag-5/5(q0)
  lag-6/6(q1_out) -> lag-5/6(q1)
  lag-6/7(q2_out) -> lag-5/7(q2)
  lag-6/8(q3_out) -> lag-5/8(q3)
  lag-6/9(lag_out) -> lag-5/9(lag_in)
  lag-5/1(i-1_out) -> lag-4/1(i0)
  lag-5/2(i0_out) -> lag-4/2(i1)
  lag-5/3(i1_out) -> lag-4/3(i2)
  lag-5/4(i2_out) -> lag-4/4(i3)
  lag-5/5(q0_out) -> lag-4/5(q0)
  lag-5/6(q1_out) -> lag-4/6(q1)
  lag-5/7(q2_out) -> lag-4/7(q2)
  lag-5/8(q3_out) -> lag-4/8(q3)
  lag-5/9(lag_out) -> lag-4/9(lag_in)
  lag-4/1(i-1_out) -> lag-3/1(i0)
  lag-4/2(i0_out) -> lag-3/2(i1)
  lag-4/3(i1_out) -> lag-3/3(i2)
  lag-4/4(i2_out) -> lag-3/4(i3)
  lag-4/5(q0_out) -> lag-3/5(q0)
  lag-4/6(q1_out) -> lag-3/6(q1)
  lag-4/7(q2_out) -> lag-3/7(q2)
  lag-4/8(q3_out) -> lag-3/8(q3)
  lag-4/9(lag_out) -> lag-3/9(lag_in)
  lag-3/1(i-1_out) -> lag-2/1(i0)
  lag-3/2(i0_out) -> lag-2/2(i1)
  lag-3/3(i1_out) -> lag-2/3(i2)
  lag-3/4(i2_out) -> lag-2/4(i3)
  lag-3/5(q0_out) -> lag-2/5(q0)
  lag-3/6(q1_out) -> lag-2/6(q1)
  lag-3/7(q2_out) -> lag-2/7(q2)
  lag-3/8(q3_out) -> lag-2/8(q3)
  lag-3/9(lag_out) -> lag-2/9(lag_in)
  lag-2/1(i-1_out) -> lag-1/1(i0)
  lag-2/2(i0_out) -> lag-1/2(i1)
  lag-2/3(i1_out) -> lag-1/3(i2)
  lag-2/4(i2_out) -> lag-1/4(i3)
  lag-2/5(q0_out) -> lag-1/5(q0)
  lag-2/6(q1_out) -> lag-1/6(q1)
  lag-2/7(q2_out) -> lag-1/7(q2)
  lag-2/8(q3_out) -> lag-1/8(q3)
  lag-2/9(lag_out) -> lag-1/9(lag_in)
  lag-1/1(i-1_out) -> lag0/1(i0)
  lag-1/2(i0_out) -> lag0/2(i1)
  lag-1/3(i1_out) -> lag0/3(i2)
  lag-1/4(i2_out) -> lag0/4(i3)
  lag-1/5(q0_out) -> lag0/5(q0)
  lag-1/6(q1_out) -> lag0/6(q1)
  lag-1/7(q2_out) -> lag0/7(q2)
  lag-1/8(q3_out) -> lag0/8(q3)
  lag-1/9(lag_out) -> lag0/9(lag_in)
  lag0/1(i-1_out) -> lag+1/1(i0)
  lag0/2(i0_out) -> lag+1/2(i1)
  lag0/3(i1_out) -> lag+1/3(i2)
  lag0/4(i2_out) -> lag+1/4(i3)
  lag0/5(q0_out) -> lag+1/5(q0)
  lag0/6(q1_out) -> lag+1/6(q1)
  lag0/7(q2_out) -> lag+1/7(q2)
  lag0/8(q3_out) -> lag+1/8(q3)
  lag0/9(lag_out) -> lag+1/9(lag_in)
  lag+1/1(i-1_out) -> lag+2/1(i0)
  lag+1/2(i0_out) -> lag+2/2(i1)
  lag+1/3(i1_out) -> lag+2/3(i2)
  lag+1/4(i2_out) -> lag+2/4(i3)
  lag+1/5(q0_out) -> lag+2/5(q0)
  lag+1/6(q1_out) -> lag+2/6(q1)
  lag+1/7(q2_out) -> lag+2/7(q2)
  lag+1/8(q3_out) -> lag+2/8(q3)
  lag+1/9(lag_out) -> lag+2/9(lag_in)
  lag+2/1(i-1_out) -> lag+3/1(i0)
  lag+2/2(i0_out) -> lag+3/2(i1)
  lag+2/3(i1_out) -> lag+3/3(i2)
  lag+2/4(i2_out) -> lag+3/4(i3)
  lag+2/5(q0_out) -> lag+3/5(q0)
  lag+2/6(q1_out) -> lag+3/6(q1)
  lag+2/7(q2_out) -> lag+3/7(q2)
  lag+2/8(q3_out) -> lag+3/8(q3)
  lag+2/9(lag_out) -> lag+3/9(lag_in)
  lag+3/1(i-1_out) -> lag+4/1(i0)
  lag+3/2(i0_out) -> lag+4/2(i1)
  lag+3/3(i1_out) -> lag+4/3(i2)
  lag+3/4(i2_out) -> lag+4/4(i3)
  lag+3/5(q0_out) -> lag+4/5(q0)
  lag+3/6(q1_out) -> lag+4/6(q1)
  lag+3/7(q2_out) -> lag+4/7(q2)
  lag+3/8(q3_out) -> lag+4/8(q3)
  lag+3/9(lag_out) -> lag+4/9(lag_in)
  lag+4/1(i-1_out) -> lag+5/1(i0)
  lag+4/2(i0_out) -> lag+5/2(i1)
  lag+4/3(i1_out) -> lag+5/3(i2)
  lag+4/4(i2_out) -> lag+5/4(i3)
  lag+4/5(q0_out) -> lag+5/5(q0)
  lag+4/6(q1_out) -> lag+5/6(q1)
  lag+4/7(q2_out) -> lag+5/7(q2)
  lag+4/8(q3_out) -> lag+5/8(q3)
  lag+4/9(lag_out) -> lag+5/9(lag_in)
  lag+5/1(i-1_out) -> lag+6/1(i0)
  lag+5/2(i0_out) -> lag+6/2(i1)
  lag+5/3(i1_out) -> lag+6/3(i2)
  lag+5/4(i2_out) -> lag+6/4(i3)
  lag+5/5(q0_out) -> lag+6/5(q0)
  lag+5/6(q1_out) -> lag+6/6(q1)
  lag+5/7(q2_out) -> lag+6/7(q2)
  lag+5/8(q3_out) -> lag+6/8(q3)
  lag+5/9(lag_out) -> lag+6/9(lag_in)
  lag+6/1(i-1_out) -> lag+7/1(i0)
  lag+6/2(i0_out) -> lag+7/2(i1)
  lag+6/3(i1_out) -> lag+7/3(i2)
  lag+6/4(i2_out) -> lag+7/4(i3)
  lag+6/5(q0_out) -> lag+7/5(q0)
  lag+6/6(q1_out) -> lag+7/6(q1)
  lag+6/7(q2_out) -> lag+7/7(q2)
  lag+6/8(q3_out) -> lag+7/8(q3)
  lag+6/9(lag_out) -> lag+7/9(lag_in)
  lag+7/1(i-1_out) -> lag+8/1(i0)
  lag+7/2(i0_out) -> lag+8/2(i1)
  lag+7/3(i1_out) -> lag+8/3(i2)
  lag+7/4(i2_out) -> lag+8/4(i3)
  lag+7/5(q0_out) -> lag+8/5(q0)
  lag+7/6(q1_out) -> lag+8/6(q1)
  lag+7/7(q2_out) -> lag+8/7(q2)
  lag+7/8(q3_out) -> lag+8/8(q3)
  lag+7/9(lag_out) -> lag+8/9(lag_in)
  lag+8/1(i-1_out) -> lag+9/1(i0)
  lag+8/2(i0_out) -> lag+9/2(i1)
  lag+8/3(i1_out) -> lag+9/3(i2)
  lag+8/4(i2_out) -> lag+9/4(i3)
  lag+8/5(q0_out) -> lag+9/5(q0)
  lag+8/6(q1_out) -> lag+9/6(q1)
  lag+8/7(q2_out) -> lag+9/7(q2)
  lag+8/8(q3_out) -> lag+9/8(q3)
  lag+8/9(lag_out) -> lag+9/9(lag_in)
  lag+9/1(i-1_out) -> lag+10/1(i0)
  lag+9/2(i0_out) -> lag+10/2(i1)
  lag+9/3(i1_out) -> lag+10/3(i2)
  lag+9/4(i2_out) -> lag+10/4(i3)
  lag+9/5(q0_out) -> lag+10/5(q0)
  lag+9/6(q1_out) -> lag+10/6(q1)
  lag+9/7(q2_out) -> lag+10/7(q2)
  lag+9/8(q3_out) -> lag+10/8(q3)
  lag+9/9(lag_out) -> lag+10/9(lag_in)
  lag+10/1(i-1_out) -> lag+11/1(i0)
  lag+10/2(i0_out) -> lag+11/2(i1)
  lag+10/3(i1_out) -> lag+11/3(i2)
  lag+10/4(i2_out) -> lag+11/4(i3)
  lag+10/5(q0_out) -> lag+11/5(q0)
  lag+10/6(q1_out) -> lag+11/6(q1)
  lag+10/7(q2_out) -> lag+11/7(q2)
  lag+10/8(q3_out) -> lag+11/8(q3)
  lag+10/9(lag_out) -> lag+11/9(lag_in)
  lag+11/1(i-1_out) -> lag+12/1(i0)
  lag+11/2(i0_out) -> lag+12/2(i1)
  lag+11/3(i1_out) -> lag+12/3(i2)
  lag+11/4(i2_out) -> lag+12/4(i3)
  lag+11/5(q0_out) -> lag+12/5(q0)
  lag+11/6(q1_out) -> lag+12/6(q1)
  lag+11/7(q2_out) -> lag+12/7(q2)
  lag+11/8(q3_out) -> lag+12/8(q3)
  lag+11/9(lag_out) -> lag+12/9(lag_in)
  lag+12/1(i-1_out) -> lag+13/1(i0)
  lag+12/2(i0_out) -> lag+13/2(i1)
  lag+12/3(i1_out) -> lag+13/3(i2)
  lag+12/4(i2_out) -> lag+13/4(i3)
  lag+12/5(q0_out) -> lag+13/5(q0)
  lag+12/6(q1_out) -> lag+13/6(q1)
  lag+12/7(q2_out) -> lag+13/7(q2)
  lag+12/8(q3_out) -> lag+13/8(q3)
  lag+12/9(lag_out) -> lag+13/9(lag_in)
  lag+13/1(i-1_out) -> lag+14/1(i0)
  lag+13/2(i0_out) -> lag+14/2(i1)
  lag+13/3(i1_out) -> lag+14/3(i2)
  lag+13/4(i2_out) -> lag+14/4(i3)
  lag+13/5(q0_out) -> lag+14/5(q0)
  lag+13/6(q1_out) -> lag+14/6(q1)
  lag+13/7(q2_out) -> lag+14/7(q2)
  lag+13/8(q3_out) -> lag+14/8(q3)
  lag+13/9(lag_out) -> lag+14/9(lag_in)
  lag+14/1(i-1_out) -> lag+15/1(i0)
  lag+14/2(i0_out) -> lag+15/2(i1)
  lag+14/3(i1_out) -> lag+15/3(i2)
  lag+14/4(i2_out) -> lag+15/4(i3)
  lag+14/5(q0_out) -> lag+15/5(q0)
  lag+14/6(q1_out) -> lag+15/6(q1)
  lag+14/7(q2_out) -> lag+15/7(q2)
  lag+14/8(q3_out) -> lag+15/8(q3)
  lag+14/9(lag_out) -> lag+15/9(lag_in)
  lag+15/1(i-1_out) -> term0/1
  lag+15/2(i0_out) -> term1/1
  lag+15/3(i1_out) -> term2/1
  lag+15/4(i2_out) -> term3/1
  lag+15/5(q0_out) -> term4/1
  lag+15/6(q1_out) -> term5/1
  lag+15/7(q2_out) -> term6/1
  lag+15/8(q3_out) -> term7/1
  lag+15/9(lag_out) -> lag_slice/1
  lag_slice/1 -> uncram/1(In)
  sync/1 -> stream_vacc/1(sync)
  uncram/1(Out1) -> stream_vacc/2("[0-0]")
  uncram/2(Out2) -> stream_vacc/3("[1-1]")
  uncram/3(Out3) -> stream_vacc/4("[2-2]")
  uncram/4(Out4) -> stream_vacc/5("[3-3]")
  uncram/5(Out5) -> stream_vacc/6("[4-4]")
  uncram/6(Out6) -> stream_vacc/7("[5-5]")
  uncram/7(Out7) -> stream_vacc/8("[6-6]")
  uncram/8(Out8) -> stream_vacc/9("[7-7]")
  uncram/9(Out9) -> stream_vacc/10("[8-8]")
  uncram/10(Out10) -> stream_vacc/11("[9-9]")
  uncram/11(Out11) -> stream_vacc/12("[10-10]")
  uncram/12(Out12) -> stream_vacc/13("[11-11]")
  uncram/13(Out13) -> stream_vacc/14("[12-12]")
  uncram/14(Out14) -> stream_vacc/15("[13-13]")
  uncram/15(Out15) -> stream_vacc/16("[14-14]")
  uncram/16(Out16) -> stream_vacc/17("[15-15]")
  uncram/17(Out17) -> stream_vacc/18("[16-16]")
  uncram/18(Out18) -> stream_vacc/19("[17-17]")
  uncram/19(Out19) -> stream_vacc/20("[18-18]")
  uncram/20(Out20) -> stream_vacc/21("[19-19]")
  uncram/21(Out21) -> stream_vacc/22("[20-20]")
  uncram/22(Out22) -> stream_vacc/23("[21-21]")
  uncram/23(Out23) -> stream_vacc/24("[22-22]")
  uncram/24(Out24) -> stream_vacc/25("[23-23]")
  uncram/25(Out25) -> stream_vacc/26("[24-24]")
  uncram/26(Out26) -> stream_vacc/27("[25-25]")
  uncram/27(Out27) -> stream_vacc/28("[26-26]")
  uncram/28(Out28) -> stream_vacc/29("[27-27]")
  uncram/29(Out29) -> stream_vacc/30("[28-28]")
  uncram/30(Out30) -> stream_vacc/31("[29-29]")
  uncram/31(Out31) -> stream_vacc/32("[30-30]")
  uncram/32(Out32) -> stream_vacc/33("[31-31]")
  stream_vacc/1(sync_out) -> sync_out/1
  stream_vacc/2(valid) -> valid/1
  stream_vacc/3("[n+0]") -> "[n+0]"/1
